simulink model "movingAvg"  (R2020b)
settings: Solver=FixedStepAuto  StartTime=0.0  StopTime=0.02  FixedStep=1e-5  RelTol=1e-3
settings Model: Creator=Kasper Laustsen  LastModifiedBy=Kasper Laustsen
settings SFSimCC: SimCustomHeaderCode="#include \"movingAvg.h\""  SimUserSources=movingAvg.c

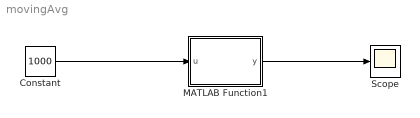
== system movingAvg ==
  Constant : Constant  Value=1000  SampleTime=-1
  MATLAB Function1 : MATLAB Function  TreatAsAtomicUnit=on
  Scope : Scope
  wires:
  Constant/1 -> MATLAB Function1/1(u)
  MATLAB Function1/1(y) -> Scope/1

== matlab function movingAvg/MATLAB Function1 ==
  data: u input; y output
function y = callingMovingAvg(u)
coder.updateBuildInfo('addSourceFiles','movingAvg.c');
coder.cinclude('movingAvg.h');

y = 0.0;
y = coder.ceval('movingAvg',u);
